simulink model "quadcopter_swarm_final_solution"  (R2023b)
settings: Solver=ode3  StartTime=0  StopTime=inf  FixedStep=0.005  RelTol=1e-3  EnableMultiTasking=on
values from neighbouring files (symbols this model uses):
  angle_outer_max = 60    [1nrx_dot.mat]    (also in 1nrxdrones_dot.mat; collision_avoidance_POS.mat; collision_avoidance_headonfix_POS.mat; collision_test.mat)
  F_e_g = [0 0 39.28]    [1nrx_dot.mat]    (also in 1nrxdrones_dot.mat; collision_avoidance_POS.mat; collision_avoidance_headonfix_POS.mat; collision_test.mat)
  g = 9.82    [1nrx_dot.mat]    (also in 1nrxdrones_dot.mat; collision_avoidance_POS.mat; collision_avoidance_headonfix_POS.mat; collision_test.mat)
  I_C = [0.5  0  0; 0  0.5  0; 0  0  1]    [1nrx_dot.mat]    (also in 1nrxdrones_dot.mat; collision_avoidance_POS.mat; collision_avoidance_headonfix_POS.mat; collision_test.mat)
  in_D = 20    [1nrx_dot.mat]    (also in 1nrxdrones_dot.mat; collision_avoidance_POS.mat; collision_avoidance_headonfix_POS.mat; collision_test.mat)
  in_I = 0    [1nrx_dot.mat]    (also in 1nrxdrones_dot.mat; collision_avoidance_POS.mat; collision_avoidance_headonfix_POS.mat; collision_test.mat)
  in_P = 20    [1nrx_dot.mat]    (also in 1nrxdrones_dot.mat; collision_avoidance_POS.mat; collision_avoidance_headonfix_POS.mat; collision_test.mat)
  in_thrust_D = 30    [1nrx_dot.mat]    (also in 1nrxdrones_dot.mat; collision_avoidance_POS.mat; collision_avoidance_headonfix_POS.mat; collision_test.mat)
  in_thrust_I = 0    [1nrx_dot.mat]    (also in 1nrxdrones_dot.mat; collision_avoidance_POS.mat; collision_avoidance_headonfix_POS.mat; collision_test.mat)
  in_thrust_P = 10    [1nrx_dot.mat]    (also in 1nrxdrones_dot.mat; collision_avoidance_POS.mat; collision_avoidance_headonfix_POS.mat; collision_test.mat)
  L = [4 -1 -1 -1 -1 0 -1 4 -1 -1 -1 0 ... (36 elements, 6x6)]    [1nrx_dot.mat]    (also in 1nrxdrones_dot.mat; collision_avoidance_POS.mat; collision_avoidance_headonfix_POS.mat; collision_test.mat)
  m = 4    [1nrx_dot.mat]    (also in 1nrxdrones_dot.mat; collision_avoidance_POS.mat; collision_avoidance_headonfix_POS.mat; collision_test.mat)
  M_RB = [4 0 0 0 0 0 0 4 0 0 0 0 ... (36 elements, 6x6)]    [1nrx_dot.mat]    (also in 1nrxdrones_dot.mat; collision_avoidance_POS.mat; collision_avoidance_headonfix_POS.mat; collision_test.mat)
  p_0 = [5  10; 5  -5; -8  5; 5  -13; 8  8; 0  0]    [1nrx_dot.mat]    (also in 1nrxdrones_dot.mat; collision_avoidance_POS.mat; collision_avoidance_headonfix_POS.mat; collision_test.mat)
  p_d = [1  0; 4  0; -2  0; 7  0; 9  0; 0  0]    [1nrx_dot.mat]    (also in 1nrxdrones_dot.mat; collision_avoidance_POS.mat; collision_avoidance_headonfix_POS.mat; collision_test.mat)
  R_c = 3    [1nrx_dot.mat]    (also in 1nrxdrones_dot.mat; collision_avoidance_POS.mat; collision_avoidance_headonfix_POS.mat; collision_test.mat)
  r_m = 2.2    [1nrx_dot.mat]    (also in 1nrxdrones_dot.mat; collision_avoidance_POS.mat; collision_avoidance_headonfix_POS.mat; collision_test.mat)
  thrust_max = 196.4    [1nrx_dot.mat]    (also in 1nrxdrones_dot.mat; collision_avoidance_POS.mat; collision_avoidance_headonfix_POS.mat; collision_test.mat)
  V = [1 2 3 4 5 6]    [1nrx_dot.mat]    (also in 1nrxdrones_dot.mat; collision_avoidance_POS.mat; collision_avoidance_headonfix_POS.mat; collision_test.mat)
  v_angle_in_max = 60    [1nrx_dot.mat]    (also in 1nrxdrones_dot.mat; collision_avoidance_POS.mat; collision_avoidance_headonfix_POS.mat; collision_test.mat)
  w = 0.6    [1nrx_dot.mat]    (also in 1nrxdrones_dot.mat; collision_avoidance_POS.mat; collision_avoidance_headonfix_POS.mat; collision_test.mat)
  w_1 = 6    [1nrx_dot.mat]    (also in 1nrxdrones_dot.mat; collision_avoidance_POS.mat; collision_avoidance_headonfix_POS.mat; collision_test.mat)
  w_2_with_h = 2.56430849099    [1nrx_dot.mat]    (also in 1nrxdrones_dot.mat; collision_avoidance_POS.mat; collision_avoidance_headonfix_POS.mat; collision_test.mat)
libraries: simulink_extras x37, slpidlib x30, sharedtransform x27, aerolibutil x25, dspsigops x24, dspindex x13, sharedutil x5, vrlib x2
(part 7 of 7)

== system quadcopter_swarm_final_solution/Drone 5/Formatting/Euler to VR/Quaternion Normalization1 ==
  e0 : Inport
  1/2 : Gain  Gain=1/2  SaturateOnIntegerOverflow=on  OutDataTypeStr=Inherit: Same as input  ParamDataTypeStr=Inherit: Same as input
  Demux : Demux  Outputs=[1 3]
      settings: DisplayOption=none
  Mux : Mux  Inputs=2
  Product : Product  InputSameDT=on  SaturateOnIntegerOverflow=on  OutDataTypeStr=Inherit: Same as first input
  Trigonometric Function : Trigonometry
  Trigonometric Function1 : Trigonometry  Operator=cos
  e0_norm : Outport  VectorParamsAs1DForOutWhenUnconnected=off
  wires:
  e0/1 -> Demux/1
  1/2/1 -> Trigonometric Function/1, Trigonometric Function1/1
  Trigonometric Function/1 -> Product/1
  Product/1 -> Mux/2
  Mux/1 -> e0_norm/1
  Demux/1 -> 1/2/1
  Demux/2 -> Product/2
  Trigonometric Function1/1 -> Mux/1

== system quadcopter_swarm_final_solution/Drone 5/Formatting/Euler to VR/Quaternion Normalization2 ==
  e0 : Inport
  1/2 : Gain  Gain=1/2  SaturateOnIntegerOverflow=on  OutDataTypeStr=Inherit: Same as input  ParamDataTypeStr=Inherit: Same as input
  Demux : Demux  Outputs=[1 3]
      settings: DisplayOption=none
  Mux : Mux  Inputs=2
  Product : Product  InputSameDT=on  SaturateOnIntegerOverflow=on  OutDataTypeStr=Inherit: Same as first input
  Trigonometric Function : Trigonometry
  Trigonometric Function1 : Trigonometry  Operator=cos
  e0_norm : Outport  VectorParamsAs1DForOutWhenUnconnected=off
  wires:
  Trigonometric Function1/1 -> Mux/1
  Demux/2 -> Product/2
  Demux/1 -> 1/2/1
  Mux/1 -> e0_norm/1
  Product/1 -> Mux/2
  Trigonometric Function/1 -> Product/1
  1/2/1 -> Trigonometric Function1/1, Trigonometric Function/1
  e0/1 -> Demux/1

== matlab function quadcopter_swarm_final_solution/Drone 5/PID controllers/Inner-loop controllers/det minimum yaw distance ==
  data: delta_yaw input; delta_yaw_min output
function delta_yaw_min = fcn(delta_yaw)

if delta_yaw > pi
    delta_yaw_min = delta_yaw - 2*pi;
elseif delta_yaw < -pi
    delta_yaw_min = delta_yaw + 2*pi;
else
    delta_yaw_min = delta_yaw;
end

== matlab function quadcopter_swarm_final_solution/Drone 1/Quadcopter model Euler/rigid-body dynamics/MATLAB Function ==
  data: tau input; nu_dot output; nu input; I_C input; M_RB input; m input
function nu_dot = fcn(tau,nu,I_C,M_RB,m)

omega_b_b_e = nu(4:6);

C_RB = [
    m*skew_sym(omega_b_b_e)     zeros(3)
    zeros(3)                    -skew_sym(I_C*omega_b_b_e)
];

nu_dot = inv(M_RB)*(tau - C_RB*nu);

end


function res = skew_sym(vector)

res = [
    0               -vector(3)      vector(2)
    vector(3)       0               -vector(1)
    -vector(2)     vector(1)       0
];

end

== matlab function quadcopter_swarm_final_solution/Drone 5/PID controllers/outer-loop velocity controller/MATLAB Function1 ==
  data: Deltap_e input; Deltap_b output; psi input
function Deltap_b = fcn(Deltap_e,psi)

R = [ cos(psi) , -sin(psi) ;
      sin(psi) ,  cos(psi) ];

Deltap_b = R'*Deltap_e;

== matlab function quadcopter_swarm_final_solution/Drone 5/Quadcopter model Euler/rigid-body dynamics/MATLAB Function ==
  data: tau input; nu_dot output; nu input; I_C input; M_RB input; m input
function nu_dot = fcn(tau,nu,I_C,M_RB,m)

omega_b_b_e = nu(4:6);

C_RB = [
    m*skew_sym(omega_b_b_e)     zeros(3)
    zeros(3)                    -skew_sym(I_C*omega_b_b_e)
];

nu_dot = inv(M_RB)*(tau - C_RB*nu);

end


function res = skew_sym(vector)

res = [
    0               -vector(3)      vector(2)
    vector(3)       0               -vector(1)
    -vector(2)     vector(1)       0
];

end

== matlab function quadcopter_swarm_final_solution/MATLAB Function ==
  data: A output; p input; L output; using_fixed_agent input; fully_connected input; k_nearest input; communication_distance input; balanced input; recieving_agents input; sending_agents input; disabled_edges input
function [A,L] = fcn( ...
    p,using_fixed_agent, ...
    fully_connected,k_nearest,communication_distance,balanced, ...
    recieving_agents,sending_agents,disabled_edges ...
    )

p_len = size(p,1);
drone_len = p_len-using_fixed_agent; % Without fixed agent

% Define the edge list
E = zeros((drone_len-1)*(drone_len),2);
R = zeros(drone_len ,drone_len);
num_edges = 1;
if fully_connected
    for i=1:drone_len 
        for j = 1:drone_len 
            if not(i == j)
                E(num_edges,:) = [i,j];
                num_edges = num_edges + 1;
            end
        end
    end
elseif communication_distance > 0
    % Define edges using min distance between vertices
    % Get min distance from drone i to all other drones
    for i=1:drone_len 
        for j=1:drone_len 
            if not(i == j)
                R(i,j) = norm(p(i,:) - p(j,:));
            else
                R(i,j) = inf;
            end
        end
    end
    R_min = mink(R,k_nearest,1);
    for i=1:drone_len 
        num_conn = 0;
        for j = 1:drone_len 
            if num_conn >= k_nearest
                break
            end
            if not(i == j) && R(i,j) <= R_min(k_nearest,i) && R(i,j) <= communication_distance
                num_conn = num_conn + 1;
                E(num_edges,:) = [i,j];
                num_edges = num_edges + 1;
                if balanced
                    E(num_edges,:) = [j,i];
                    num_edges = num_edges + 1;
                end
            end
        end
    end
else
    % Define edges using min distance between vertices
    % Get min distance from drone i to all other drones
    for i=1:drone_len 
        for j=1:drone_len 
            if not(i == j)
                R(i,j) = norm(p(i,:) - p(j,:));
            else
                R(i,j) = inf;
            end
        end
    end
    R_min = mink(R,k_nearest,1);
    for i=1:drone_len 
        num_conn = 0;
        for j = 1:drone_len 
            if num_conn >= k_nearest
                break
            end
            if not(i == j) && R(i,j) <= R_min(k_nearest,i)
                num_conn = num_conn + 1;
                E(num_edges,:) = [i,j];
                num_edges = num_edges + 1;
                if balanced
                    E(num_edges,:) = [j,i];
                    num_edges = num_edges + 1;
                end
            end
        end
    end
end


% Define adjacancy matrix A based on these edges
A = zeros(p_len);
if using_fixed_agent
    for i=1:p_len
        if i == p_len %Meaning this is the fix-agent
            A(i,:) = 0;
        else
            for j = 1:p_len
                if j == p_len
                    A(i,j) = 1;
                end
                for edge = 1:(num_edges-1)
                    edge_vals = E(edge,:);
                    A(edge_vals(1),edge_vals(2)) = 1;
                end
            end
        end
    end
else
    for edge = 1:(num_edges-1)
        edge_vals = E(edge,:);
        A(edge_vals(1),edge_vals(2)) = 1;
    end
end

% Removing disconnected agents
% remove the ones that stopped recieving
for i=1:p_len
    if recieving_agents(i) == 0
        A(i,:) = 0;
    end
end
% remove the onse that stopped sending
for j=1:p_len
    if sending_agents(j) == 0
        A(:,j) = 0;
    end
end
% remove the edges that are not allowed
A = A.*(ones(p_len)-disabled_edges);


% Defining degree matrix D
D = zeros(p_len);
for i=1:p_len
    for j=1:p_len
        if not(i==j)
            D(i,i) = D(i,i) + A(i,j);
        end
    end
end


% Defnining graph Laplacian L
L = D-A;

== matlab function quadcopter_swarm_final_solution/Desired position Laplacian with Collision Avoidance and head-on collision avoidance /Swarm Velocities ==
  data: delta_p input; p_dot output; w input; L input
function p_dot = Fun1(delta_p,w,L)

p_dot = -w*tanh((1/w)*L*delta_p);

== matlab function quadcopter_swarm_final_solution/Drone 2/PID controllers/Inner-loop controllers/det minimum yaw distance ==
  data: delta_yaw input; delta_yaw_min output
function delta_yaw_min = fcn(delta_yaw)

if delta_yaw > pi
    delta_yaw_min = delta_yaw - 2*pi;
elseif delta_yaw < -pi
    delta_yaw_min = delta_yaw + 2*pi;
else
    delta_yaw_min = delta_yaw;
end

== matlab function quadcopter_swarm_final_solution/Desired position Laplacian with Collision Avoidance and head-on collision avoidance /Collision Avoidance ==
  data: p input; p_dot_2 output; w_2 input; r_m input; dist output; R_c input
function [p_dot_2, dist] = Fun2(p, w_2, r_m, R_c)

n_drones = size(p,1) -1;
n_dim = size(p,2);

p_dot_2 = zeros(n_drones + 1,n_dim);
dist = zeros(n_drones + 1,1);


for i = 1:(n_drones)
    for j = 1:(n_drones)
        if not(i == j)
            d_ij = sqrt((p(i,1)-p(j,1))^2+(p(i,2)-p(j,2))^2);
            dist(i) = d_ij;
            if d_ij < R_c
                p_dot_2(i,:) = p_dot_2(i,:) + w_2*(atan2(d_ij^2-r_m^2,1) - atan2(d_ij^2+pi^2,1))*(p(i,:)-p(j,:))/d_ij; 
            end
        end
    end
end

end

== matlab function quadcopter_swarm_final_solution/Desired position Laplacian with Collision Avoidance and head-on collision avoidance /Head On Collision Solver ==
  data: fun2 input; p_dot_h output
function p_dot_h = h(fun2)

fun2x = fun2(:,1);
fun2y = fun2(:,2);


p_dot_h = 0.5*[fun2y,fun2x];

== matlab function quadcopter_swarm_final_solution/Drone 1/PID controllers/Inner-loop controllers/det minimum yaw distance ==
  data: delta_yaw input; delta_yaw_min output
function delta_yaw_min = fcn(delta_yaw)

if delta_yaw > pi
    delta_yaw_min = delta_yaw - 2*pi;
elseif delta_yaw < -pi
    delta_yaw_min = delta_yaw + 2*pi;
else
    delta_yaw_min = delta_yaw;
end

== matlab function quadcopter_swarm_final_solution/Drone 2/PID controllers/outer-loop velocity controller/MATLAB Function1 ==
  data: Deltap_e input; Deltap_b output; psi input
function Deltap_b = fcn(Deltap_e,psi)

R = [ cos(psi) , -sin(psi) ;
      sin(psi) ,  cos(psi) ];

Deltap_b = R'*Deltap_e;

== matlab function quadcopter_swarm_final_solution/Drone 1/PID controllers/outer-loop velocity controller/MATLAB Function1 ==
  data: Deltap_e input; Deltap_b output; psi input
function Deltap_b = fcn(Deltap_e,psi)

R = [ cos(psi) , -sin(psi) ;
      sin(psi) ,  cos(psi) ];

Deltap_b = R'*Deltap_e;

== matlab function quadcopter_swarm_final_solution/Drone 2/Quadcopter model Euler/rigid-body dynamics/MATLAB Function ==
  data: tau input; nu_dot output; nu input; I_C input; M_RB input; m input
function nu_dot = fcn(tau,nu,I_C,M_RB,m)

omega_b_b_e = nu(4:6);

C_RB = [
    m*skew_sym(omega_b_b_e)     zeros(3)
    zeros(3)                    -skew_sym(I_C*omega_b_b_e)
];

nu_dot = inv(M_RB)*(tau - C_RB*nu);

end


function res = skew_sym(vector)

res = [
    0               -vector(3)      vector(2)
    vector(3)       0               -vector(1)
    -vector(2)     vector(1)       0
];

end

== matlab function quadcopter_swarm_final_solution/Drone 3/PID controllers/Inner-loop controllers/det minimum yaw distance ==
  data: delta_yaw input; delta_yaw_min output
function delta_yaw_min = fcn(delta_yaw)

if delta_yaw > pi
    delta_yaw_min = delta_yaw - 2*pi;
elseif delta_yaw < -pi
    delta_yaw_min = delta_yaw + 2*pi;
else
    delta_yaw_min = delta_yaw;
end

== matlab function quadcopter_swarm_final_solution/Drone 3/PID controllers/outer-loop velocity controller/MATLAB Function1 ==
  data: Deltap_e input; Deltap_b output; psi input
function Deltap_b = fcn(Deltap_e,psi)

R = [ cos(psi) , -sin(psi) ;
      sin(psi) ,  cos(psi) ];

Deltap_b = R'*Deltap_e;

== matlab function quadcopter_swarm_final_solution/Drone 3/Quadcopter model Euler/rigid-body dynamics/MATLAB Function ==
  data: tau input; nu_dot output; nu input; I_C input; M_RB input; m input
function nu_dot = fcn(tau,nu,I_C,M_RB,m)

omega_b_b_e = nu(4:6);

C_RB = [
    m*skew_sym(omega_b_b_e)     zeros(3)
    zeros(3)                    -skew_sym(I_C*omega_b_b_e)
];

nu_dot = inv(M_RB)*(tau - C_RB*nu);

end


function res = skew_sym(vector)

res = [
    0               -vector(3)      vector(2)
    vector(3)       0               -vector(1)
    -vector(2)     vector(1)       0
];

end

== matlab function quadcopter_swarm_final_solution/Drone 4/PID controllers/Inner-loop controllers/det minimum yaw distance ==
  data: delta_yaw input; delta_yaw_min output
function delta_yaw_min = fcn(delta_yaw)

if delta_yaw > pi
    delta_yaw_min = delta_yaw - 2*pi;
elseif delta_yaw < -pi
    delta_yaw_min = delta_yaw + 2*pi;
else
    delta_yaw_min = delta_yaw;
end

== matlab function quadcopter_swarm_final_solution/Drone 4/PID controllers/outer-loop velocity controller/MATLAB Function1 ==
  data: Deltap_e input; Deltap_b output; psi input
function Deltap_b = fcn(Deltap_e,psi)

R = [ cos(psi) , -sin(psi) ;
      sin(psi) ,  cos(psi) ];

Deltap_b = R'*Deltap_e;

== matlab function quadcopter_swarm_final_solution/Drone 4/Quadcopter model Euler/rigid-body dynamics/MATLAB Function ==
  data: tau input; nu_dot output; nu input; I_C input; M_RB input; m input
function nu_dot = fcn(tau,nu,I_C,M_RB,m)

omega_b_b_e = nu(4:6);

C_RB = [
    m*skew_sym(omega_b_b_e)     zeros(3)
    zeros(3)                    -skew_sym(I_C*omega_b_b_e)
];

nu_dot = inv(M_RB)*(tau - C_RB*nu);

end


function res = skew_sym(vector)

res = [
    0               -vector(3)      vector(2)
    vector(3)       0               -vector(1)
    -vector(2)     vector(1)       0
];

end
